simulink library "Heart_Signal_Processing_Library"  (R2021b)
settings: Solver=VariableStepAuto  StartTime=0.0  StopTime=10.0  RelTol=1e-3
undefined symbols (not defined in the file): sampleTime
libraries: coefficientsOfTunableBandpassFilter x10, simulink x2, dspindex x1
Description:
  | This library contains the subsystems that can be used to create the Pan-Tompkin algorithm and the Subsystems necessary for Non_invasive
  | Blood Pressure Signal Processing.
  | 
  | The lowpassFilter and the highpassFilter can be cascaded to create a first-order bandpass filter,
  | similar to that of the one used in the Pan-Tompkin Algorithm.
  | 
  | The tunableBandpassFilter is a second order bandpass filter with tunable quality factor and center frequency settings,
  | that can be used as a drop-in replacement to the cascaded lowpassFilter and highpassFilter.
  | 
  | The purpose of the bandpass filter is to attenuate the lower frequency and higher frequency components of the ecg signal, while
  | allowing the frequency of the QRS signal component to pass as an output.
  | 
  | The derivative filter is meant to be placed after a bandpass filter, and is designed to further amplify the QRS wave magnitude
  | since the QRS wave's rate of change is much larger than that of the remaining frequency components' magnitude.
  | 
  | The movingAvg (moving average) filter is designed to be placed after a squaring function (which should have been placed right after the derivative filter),
  | and is a done so that the area where the QRS is present is expanded in regards to timespan.
  | 
  | The tresholdQRS is a block that is used at two different locations in the Pan-Tompkin Algorithm.
  | The first location this block is used is right after the chosen bandpass filter and right before a delay that is placed to sync the output
  | of the first thresholdQRS with that of the second thresholdQRS. The signal that comes out of the delay is placed through an AND gate
  | with the signal that comes out of the second delay. This results in a detected QRS. The second thresholdQRS is to be placed after the movingAvg.
  | Independelty, both thresholdQRS output a possible QRS detection as a value of 1, these values, especially the one out of the first threshold,
  | are likely to contain false positives which is why they are synced and compared using AND logic.
  | 
  | The bandpassStartupTimer acts as a temporary buffer between the first 0.5 seconds of the chosen bandpass and the derivative filters.
  | Outputs 0 prior to the 0.5 seconds, and then passes the bandpass filter otuput into the derivative filter after the 0.5 seconds. This component
  | helps eliminate the possiblility of false negatives caused by an abnormally high signal threshold initial values that could occur prior to 0.5 seconds.
  | 
  | The QRS_startupTimer acts as a temporary buffer right before the final QRS detection output. Any value prior to 3.6 seconds is set to 0.
  | After 3.6 seconds, the intended confirmed QRS values are allowed through. This buffer helps prevent false positives caused during the
  | initialization of the system prior to 3.6 seconds. Note: The last known false positives occur before 2 seconds, but 3.6 seconds allows for an
  | addtional 80% margin of error.
settings Model: Creator=wallyproenza  LastModifiedBy=wallyproenza

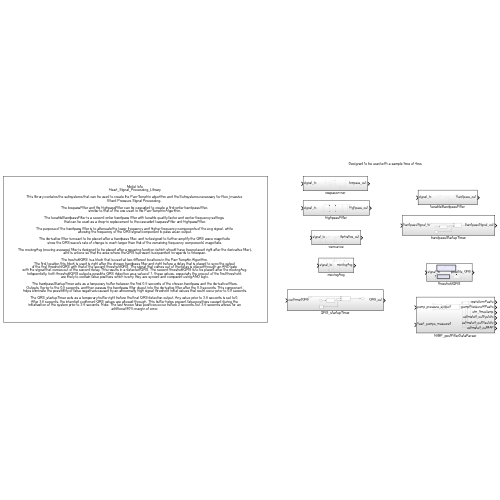
[thumbnail: Simulink's stored preview of the top-level diagram]
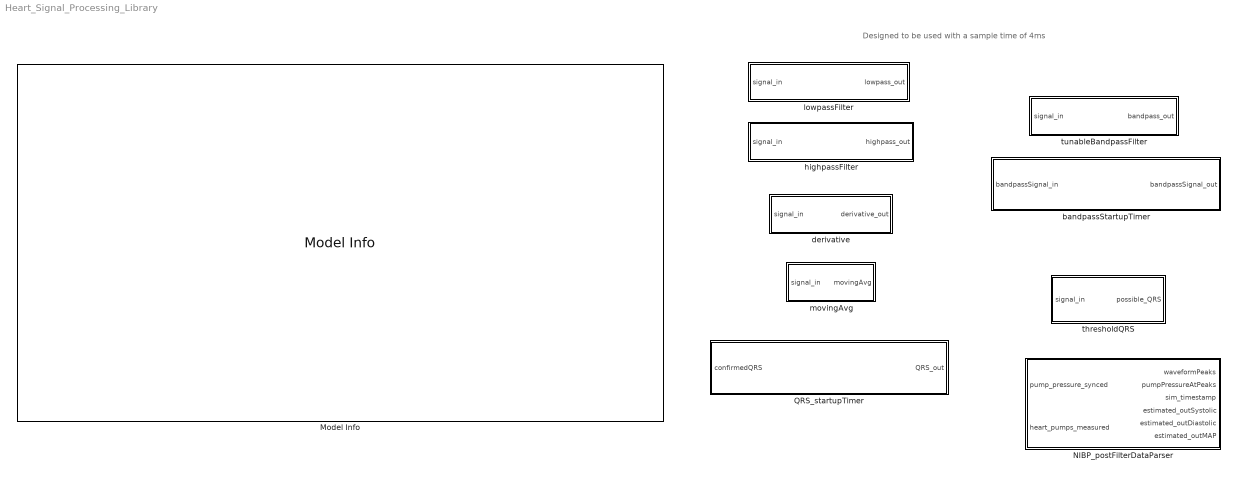
== system Heart_Signal_Processing_Library ==
  note: Designed to be used with a sample time of 4ms
  Model Info : simulink/Model-Wide Utilities/Model Info  Frame=on  DisplayStringWithTags=|  HorizontalTextAlignment=Center  LeftAlignmentValue=0.5
      | Model Info
      | %<ModelName>
      | 
      | %<Description>
  NIBP_postFilterDataParser : Subsystem
  QRS_startupTimer : Subsystem  Description=|
      | The QRS_startupTimer acts as a temporary buffer right before the final QRS detection output. Any value prior to 3.6 seconds is set to 0. 
      | After 3.6 seconds, the intended confirmed QRS values are allowed through. This buffer helps prevent false positives caused during the 
      | initialization of the system prior to 3.6 seconds. Note: The last known false positives occur before 2 seconds, but 3.6 seconds allows for an 
      | addtional 80% margin of error.
  bandpassStartupTimer : Subsystem  Description=|
      | The bandpassStartupTimer acts as a temporary buffer between the first 0.5 seconds of the chosen bandpass and the derivative filters.
      | Outputs 0 prior to the 0.5 seconds, and then passes the bandpass filter otuput into the derivative filter after the 0.5 seconds. This component 
      | helps eliminate the possiblility of false negatives caused by an abnormally high signal threshold initial values that could occur prior to 0.5 seconds.
  derivative : Subsystem  Description=|
      | The derivative filter is meant to be placed after a bandpass filter, and is designed to further amplify the QRS wave 
      | magnitude since the QRS wave's rate of change is much larger than that of the remaining frequency components' 
      | magnitude.
  highpassFilter : Subsystem  Description=|
      | Highpass filter described by the following difference equation:
      | y[n] = - (1/32)*x[n] + x[n-16] - x [n - 17] + (1/32)*x[n-32] + y[n-1]
  lowpassFilter : Subsystem  Description=|
      | Lowpass filter described by the below difference equation:
      | y[n] = (1/36)*(x[n] - 2x[n-6] + x[n-12]) + 2y[n-1] - y[n-2]
  movingAvg : Subsystem  Description=|
      | The movingAvg (moving average) filter is designed to be placed after a squaring function (which should have been placed right after the derivative filter),
      | and is a done so that the area where the QRS is present is expanded in regards to timespan. 
      | 
      | The moving average filter takes the average of the most recent 38 samples. This is implemented with a running sum of the most recent 38 samples 
      | with the 39th oldest sample subtracted whenever a new sample is introduced to the sum. Then the sum is divided by 38.
  thresholdQRS : Subsystem  Description=|
      | The tresholdQRS is a block that is used at two different locations in the Pan-Tompkin Algorithm. 
      | The first location this block is used is right after the chosen bandpass filter and right before a delay that is placed to sync the output 
      | of the first thresholdQRS with that of the second thresholdQRS. The signal that comes out of the delay is placed through an AND gate 
      | with the signal that comes out of the second delay. This results in a detected QRS. The second thresholdQRS is to be placed after the movingAvg.
      | Independelty, both thresholdQRS output a possible QRS detection as a value of 1, these values, especially the one out of the first threshold, 
      | are likely to contain false positives which is why they are synced and compared using AND logic.
  tunableBandpassFilter : Subsystem  Description=|
      | Bandpass Filter described by the following diference equation in terms of tunable centerFrequency f_o and qualityFactor Q:
      | y[n]=1/(250*10^3+π*10^3*f_o/Q  +4π^2 f_o^2 )*(π*10^3*f_o/Q x[n]  − π*10^3*f_o/Q x[n−2]  −(250*10^3−π*10^3*f_o/Q  +4π^2 f_o^2 )y[n−2]−2*(4π^2 f_o^2  −250*10^3 )y[n−1])
      | 
      | 
      | For simplicity, let constants A, B, and C be subsystems that contain the corresponding defintiions of the coefficients:
      | y[n] = 1/(A+ B + C ) * {Bx[n]  − Bx[n−2]  − (A − B + C )y[n−2]− 2*(C  − A)y[n−1]}
      | 
      | where,
      | A = 250*10^3
      | B = π*10^3*f_o/Q  
      | C = 4π^2 f_o^2

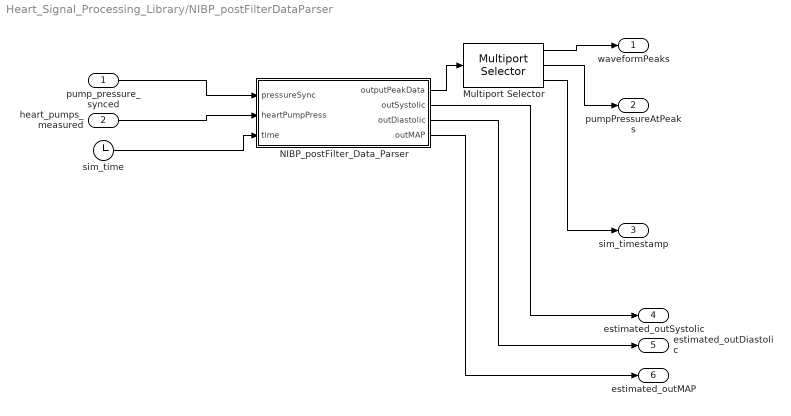
== system Heart_Signal_Processing_Library/NIBP_postFilterDataParser ==
  pump_pressure_synced : Inport
  heart_pumps_measured : Inport  Port=2
  Multiport Selector : dspindex/Multiport Selector  rowsOrCols=Columns  idxCellArray={ 1, 2, 3}  idxErrMode=Clip Index
  NIBP_postFilter_Data_Parser : MATLAB Function  TreatAsAtomicUnit=on
  sim_time : Clock
  waveformPeaks : Outport
  pumpPressureAtPeaks : Outport  Port=2
  sim_timestamp : Outport  Port=3
  estimated_outSystolic : Outport  Port=4
  estimated_outDiastolic : Outport  Port=5
  estimated_outMAP : Outport  Port=6
  wires:
  heart_pumps_measured/1 -> NIBP_postFilter_Data_Parser/2(heartPumpPress)
  Multiport Selector/3 -> sim_timestamp/1
  NIBP_postFilter_Data_Parser/3(outDiastolic) -> estimated_outDiastolic/1
  NIBP_postFilter_Data_Parser/4(outMAP) -> estimated_outMAP/1
  pump_pressure_synced/1 -> NIBP_postFilter_Data_Parser/1(pressureSync)
  Multiport Selector/1 -> waveformPeaks/1
  sim_time/1 -> NIBP_postFilter_Data_Parser/3(time)
  NIBP_postFilter_Data_Parser/2(outSystolic) -> estimated_outSystolic/1
  Multiport Selector/2 -> pumpPressureAtPeaks/1
  NIBP_postFilter_Data_Parser/1(outputPeakData) -> Multiport Selector/1

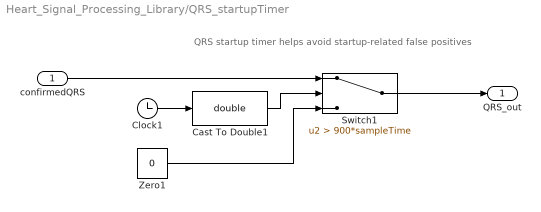
== system Heart_Signal_Processing_Library/QRS_startupTimer ==
  note: QRS startup timer helps avoid startup-related false positives
  confirmedQRS : Inport
  Cast To Double1 : DataTypeConversion  OutDataTypeStr=double
  Clock1 : Clock
  Switch1 : Switch  Criteria=u2 > Threshold  Threshold=900*sampleTime
  Zero1 : Constant  Value=0  OutDataTypeStr=Inherit: Inherit via back propagation
  QRS_out : Outport
  wires:
  confirmedQRS/1 -> Switch1/1
  Zero1/1 -> Switch1/3
  Cast To Double1/1 -> Switch1/2
  Switch1/1 -> QRS_out/1
  Clock1/1 -> Cast To Double1/1

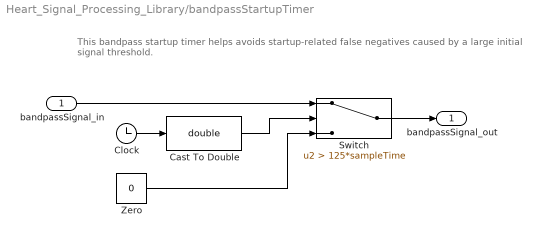
== system Heart_Signal_Processing_Library/bandpassStartupTimer ==
  note: This bandpass startup timer helps avoids startup-related false negatives
      | caused by a large initial signal threshold.
  bandpassSignal_in : Inport
  Cast To Double : DataTypeConversion  OutDataTypeStr=double
  Clock : Clock
  Switch : Switch  Criteria=u2 > Threshold  Threshold=125*sampleTime
  Zero : Constant  Value=0  OutDataTypeStr=Inherit: Inherit via back propagation
  bandpassSignal_out : Outport
  wires:
  Cast To Double/1 -> Switch/2
  Switch/1 -> bandpassSignal_out/1
  bandpassSignal_in/1 -> Switch/1
  Zero/1 -> Switch/3
  Clock/1 -> Cast To Double/1

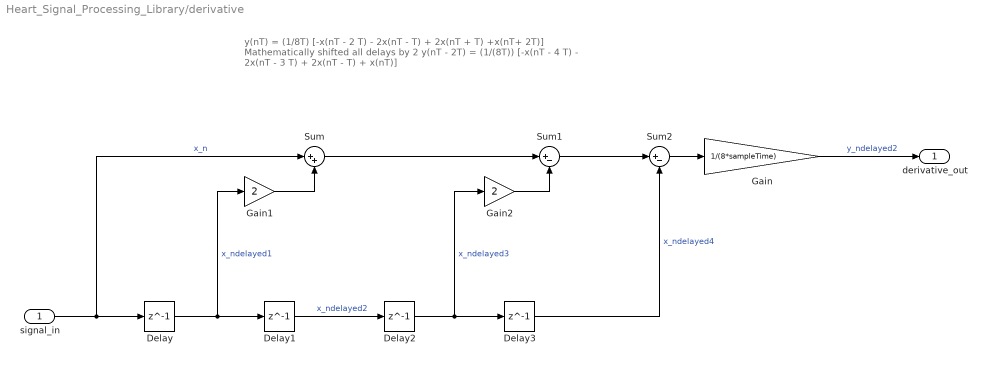
== system Heart_Signal_Processing_Library/derivative ==
  note: y(nT) = (1/8T) [-x(nT - 2 T) - 2x(nT - T) + 2x(nT + T) +x(nT+ 2T)]
      |
      | Mathematically shifted all delays by 2
      |
      | y(nT - 2T) = (1/(8T)) [-x(nT - 4 T) - 2x(nT - 3 T) + 2x(nT - T) + x(nT)]
  signal_in : Inport
  Delay{,1..3} (4 alike) : Delay  DelayLength=1  InitialCondition=0
  Gain : Gain  Gain=1/(8*sampleTime)
  Gain1 : Gain  Gain=2
  Gain2 : Gain  Gain=2
  Sum : Sum  Inputs=|++
  Sum1 : Sum  Inputs=|+-
  Sum2 : Sum  Inputs=|+-
  derivative_out : Outport
  wires:
  Gain/1 -> derivative_out/1  "y_ndelayed2"
  signal_in/1 -> Sum/1, Delay/1  "x_n"
  Delay/1 -> Gain1/1, Delay1/1  "x_ndelayed1"
  Delay1/1 -> Delay2/1  "x_ndelayed2"
  Delay2/1 -> Gain2/1, Delay3/1  "x_ndelayed3"
  Delay3/1 -> Sum2/2  "x_ndelayed4"
  Gain1/1 -> Sum/2
  Gain2/1 -> Sum1/2
  Sum/1 -> Sum1/1
  Sum1/1 -> Sum2/1
  Sum2/1 -> Gain/1

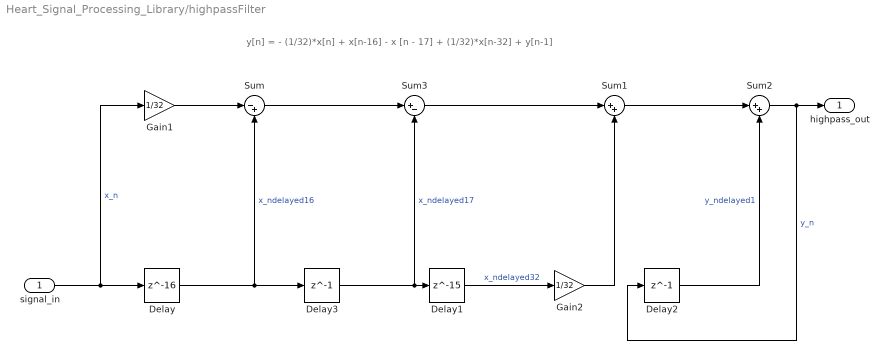
== system Heart_Signal_Processing_Library/highpassFilter ==
  note: y[n] = - (1/32)*x[n] + x[n-16] - x [n - 17] + (1/32)*x[n-32] + y[n-1]
  signal_in : Inport
  Delay : Delay  DelayLength=16  InitialCondition=0
  Delay1 : Delay  DelayLength=15  InitialCondition=0
  Delay2 : Delay  DelayLength=1  InitialCondition=0
  Delay3 : Delay  DelayLength=1  InitialCondition=0
  Gain1 : Gain  Gain=1/32
  Gain2 : Gain  Gain=1/32
  Sum : Sum  Inputs=|-+
  Sum1 : Sum  Inputs=|++
  Sum2 : Sum  Inputs=|++
  Sum3 : Sum  Inputs=|+-
  highpass_out : Outport
  wires:
  signal_in/1 -> Gain1/1, Delay/1  "x_n"
  Delay/1 -> Delay3/1, Sum/2  "x_ndelayed16"
  Delay1/1 -> Gain2/1  "x_ndelayed32"
  Sum1/1 -> Sum2/1
  Delay2/1 -> Sum2/2  "y_ndelayed1"
  Sum2/1 -> Delay2/1, highpass_out/1  "y_n"
  Gain1/1 -> Sum/1
  Delay3/1 -> Delay1/1, Sum3/2  "x_ndelayed17"
  Sum/1 -> Sum3/1
  Sum3/1 -> Sum1/1
  Gain2/1 -> Sum1/2

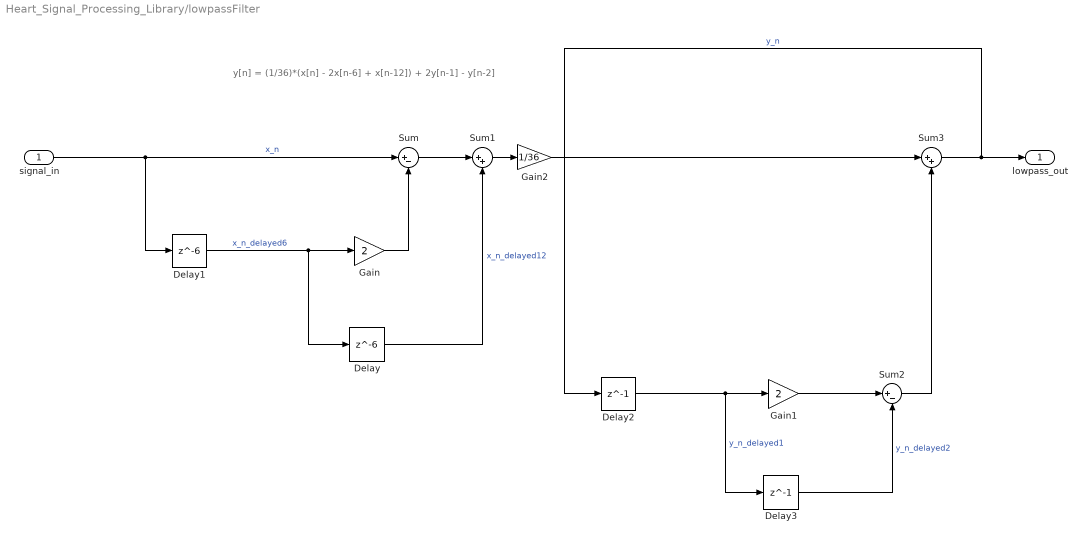
== system Heart_Signal_Processing_Library/lowpassFilter ==
  note: y[n] = (1/36)*(x[n] - 2x[n-6] + x[n-12]) + 2y[n-1] - y[n-2]
  signal_in : Inport
  Delay : Delay  DelayLength=6  InitialCondition=0
  Delay1 : Delay  DelayLength=6  InitialCondition=0
  Delay2 : Delay  DelayLength=1  InitialCondition=0
  Delay3 : Delay  DelayLength=1  InitialCondition=0
  Gain : Gain  Gain=2
  Gain1 : Gain  Gain=2
  Gain2 : Gain  Gain=1/36
  Sum : Sum  Inputs=|+-
  Sum1 : Sum  Inputs=|++
  Sum2 : Sum  Inputs=|+-
  Sum3 : Sum  Inputs=|++
  lowpass_out : Outport
  wires:
  signal_in/1 -> Delay1/1, Sum/1  "x_n"
  Delay1/1 -> Gain/1, Delay/1  "x_n_delayed6"
  Gain/1 -> Sum/2
  Delay/1 -> Sum1/2  "x_n_delayed12"
  Sum/1 -> Sum1/1
  Sum1/1 -> Gain2/1
  Delay2/1 -> Delay3/1, Gain1/1  "y_n_delayed1"
  Gain1/1 -> Sum2/1
  Delay3/1 -> Sum2/2  "y_n_delayed2"
  Sum2/1 -> Sum3/2
  Sum3/1 -> lowpass_out/1, Delay2/1  "y_n"
  Gain2/1 -> Sum3/1

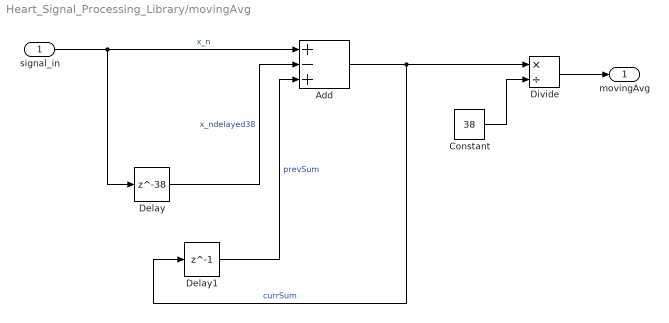
== system Heart_Signal_Processing_Library/movingAvg ==
  signal_in : Inport
  Add : Sum  Inputs=+-+
  Constant : Constant  Value=38
  Delay : Delay  DelayLength=38  InitialCondition=0
  Delay1 : Delay  DelayLength=1  InitialCondition=0
  Divide : Product  Inputs=*/
  movingAvg : Outport
  wires:
  Constant/1 -> Divide/2
  Divide/1 -> movingAvg/1
  signal_in/1 -> Delay/1, Add/1  "x_n"
  Delay/1 -> Add/2  "x_ndelayed38"
  Add/1 -> Divide/1, Delay1/1  "currSum"
  Delay1/1 -> Add/3  "prevSum"

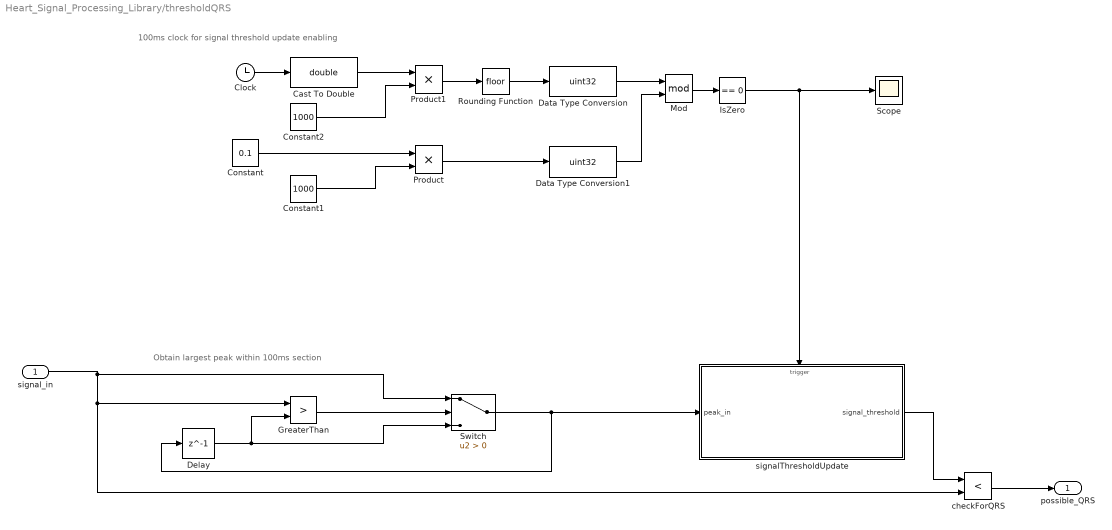
== system Heart_Signal_Processing_Library/thresholdQRS ==
  note: Obtain largest peak within 100ms section
  note: 100ms clock for signal threshold update enabling
  signal_in : Inport
  Cast To Double : DataTypeConversion  OutDataTypeStr=double
  Clock : Clock
  Constant : Constant  Value=0.1
  Constant1 : Constant  Value=1000
  Constant2 : Constant  Value=1000
  Data Type Conversion : DataTypeConversion  OutDataTypeStr=uint32
  Data Type Conversion1 : DataTypeConversion  OutDataTypeStr=uint32
  Delay : Delay  DelayLength=1  InitialCondition=0
  GreaterThan : RelationalOperator  Operator=>  OutDataTypeStr=boolean  RndMeth=Simplest
  IsZero : simulink/Logic and Bit Operations/Compare To Zero  relop===  OutDataTypeStr=boolean
  Mod : Math  Operator=mod  SaturateOnIntegerOverflow=on
  Product : Product
  Product1 : Product
  Rounding Function : Rounding
  Scope : Scope
  Switch : Switch  Criteria=u2 > Threshold
  checkForQRS : RelationalOperator  Operator=<  OutDataTypeStr=boolean  RndMeth=Simplest
  signalThresholdUpdate : Subsystem
  possible_QRS : Outport
  wires:
  signal_in/1 -> checkForQRS/2, GreaterThan/1, Switch/1
  signalThresholdUpdate/1(signal_threshold) -> checkForQRS/1
  Rounding Function/1 -> Data Type Conversion/1
  Constant/1 -> Product/1
  Product/1 -> Data Type Conversion1/1
  Constant1/1 -> Product/2
  Constant2/1 -> Product1/2
  Clock/1 -> Cast To Double/1
  Product1/1 -> Rounding Function/1
  Data Type Conversion1/1 -> Mod/2
  Data Type Conversion/1 -> Mod/1
  Mod/1 -> IsZero/1
  IsZero/1 -> signalThresholdUpdate/Trigger, Scope/1
  Cast To Double/1 -> Product1/1
  checkForQRS/1 -> possible_QRS/1
  GreaterThan/1 -> Switch/2
  Switch/1 -> Delay/1, signalThresholdUpdate/1(peak_in)
  Delay/1 -> Switch/3, GreaterThan/2

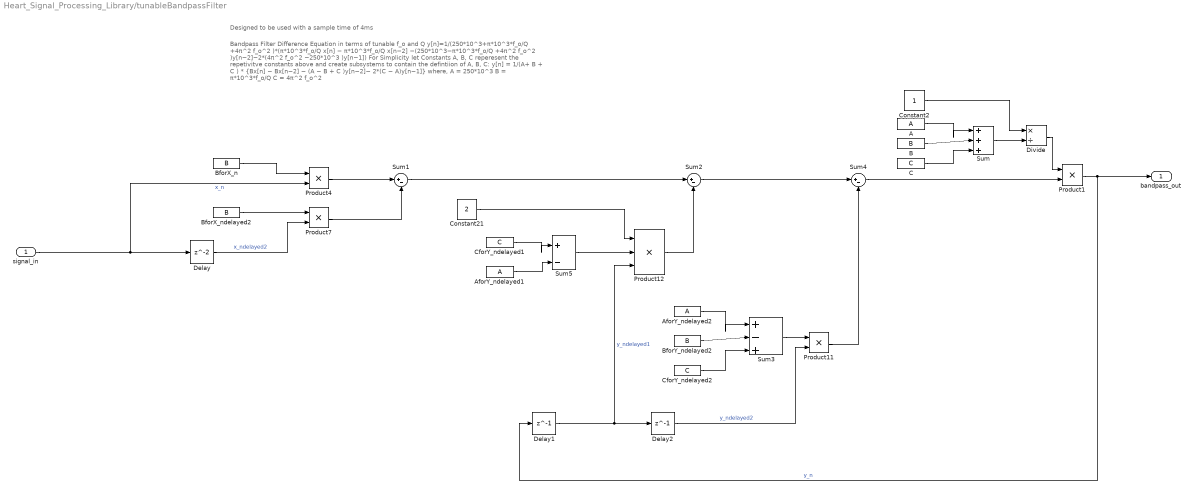
== system Heart_Signal_Processing_Library/tunableBandpassFilter ==
  note: Bandpass Filter Difference Equation in terms of tunable f_o and Q
      |
      | y[n]=1/(250*10^3+π*10^3*f_o/Q +4π^2 f_o^2 )*(π*10^3*f_o/Q x[n] − π*10^3*f_o/Q x[n−2] −(250*10^3−π*10^3*f_o/Q +4π^2 f_o^2 )y[n−2]−2*(4π^2 f_o^2 −250*10^3 )y[n−1])
      |
      | For Simplicity let Constants A, B, C reperesent the repetivitve constants above and create subsystems to contain the defintiion of A, B, C:
      |
      | y[n] = 1/(A+ B + C ) * {Bx[n] − Bx[n−2] − (A − B + C )y[n−2]− 2*(C − A)y[n−1]}
      |
      | where,
      | A = 250*10^3
      | B = π*10^3*f_o/Q
      | C = 4π^2 f_o^2
  note: Designed to be used with a sample time of 4ms
  signal_in : Inport
  A : coefficientsOfTunableBandpassFilter/A  SystemSampleTime=-1  VariantActivationTime=update diagram  Latency=0  AutoFrameSizeCalculation=off
  AforY_ndelayed1 : coefficientsOfTunableBandpassFilter/A  SystemSampleTime=-1  VariantActivationTime=update diagram  Latency=0  AutoFrameSizeCalculation=off
  AforY_ndelayed2 : coefficientsOfTunableBandpassFilter/A  SystemSampleTime=-1  VariantActivationTime=update diagram  Latency=0  AutoFrameSizeCalculation=off
  B : coefficientsOfTunableBandpassFilter/B  SystemSampleTime=-1  VariantActivationTime=update diagram  Latency=0  AutoFrameSizeCalculation=off
  BforX_n : coefficientsOfTunableBandpassFilter/B  SystemSampleTime=-1  VariantActivationTime=update diagram  Latency=0  AutoFrameSizeCalculation=off
  BforX_ndelayed2 : coefficientsOfTunableBandpassFilter/B  SystemSampleTime=-1  VariantActivationTime=update diagram  Latency=0  AutoFrameSizeCalculation=off
  BforY_ndelayed2 : coefficientsOfTunableBandpassFilter/B  SystemSampleTime=-1  VariantActivationTime=update diagram  Latency=0  AutoFrameSizeCalculation=off
  C : coefficientsOfTunableBandpassFilter/C  SystemSampleTime=-1  VariantActivationTime=update diagram  Latency=0  AutoFrameSizeCalculation=off
  CforY_ndelayed1 : coefficientsOfTunableBandpassFilter/C  SystemSampleTime=-1  VariantActivationTime=update diagram  Latency=0  AutoFrameSizeCalculation=off
  CforY_ndelayed2 : coefficientsOfTunableBandpassFilter/C  SystemSampleTime=-1  VariantActivationTime=update diagram  Latency=0  AutoFrameSizeCalculation=off
  Constant2 : Constant
  Constant21 : Constant  Value=2
  Delay : Delay  InitialCondition=0
  Delay1 : Delay  DelayLength=1  InitialCondition=0
  Delay2 : Delay  DelayLength=1  InitialCondition=0
  Divide : Product  Inputs=*/
  Product{1,4,7,11} (4 alike) : Product
  Product12 : Product  Inputs=3
  Sum : Sum  Inputs=|+++
  Sum{1..2,4..5} (4 alike) : Sum  Inputs=|+-
  Sum3 : Sum  Inputs=|+-+
  bandpass_out : Outport
  wires:
  signal_in/1 -> Product4/2, Delay/1  "x_n"
  Delay1/1 -> Product12/3, Delay2/1  "y_ndelayed1"
  Product1/1 -> Delay1/1, bandpass_out/1  "y_n"
  Constant2/1 -> Divide/1
  Sum/1 -> Divide/2
  Divide/1 -> Product1/1
  Product4/1 -> Sum1/1
  Product7/1 -> Sum1/2
  Delay/1 -> Product7/2  "x_ndelayed2"
  Sum1/1 -> Sum2/1
  Sum3/1 -> Product11/1
  Product11/1 -> Sum4/2
  Delay2/1 -> Product11/2  "y_ndelayed2"
  Sum4/1 -> Product1/2
  Sum2/1 -> Sum4/1
  Product12/1 -> Sum2/2
  Constant21/1 -> Product12/1
  Sum5/1 -> Product12/2
  A/1 -> Sum/1
  B/1 -> Sum/2
  C/1 -> Sum/3
  BforX_n/1 -> Product4/1
  BforX_ndelayed2/1 -> Product7/1
  AforY_ndelayed1/1 -> Sum5/2
  CforY_ndelayed1/1 -> Sum5/1
  AforY_ndelayed2/1 -> Sum3/1
  BforY_ndelayed2/1 -> Sum3/2
  CforY_ndelayed2/1 -> Sum3/3

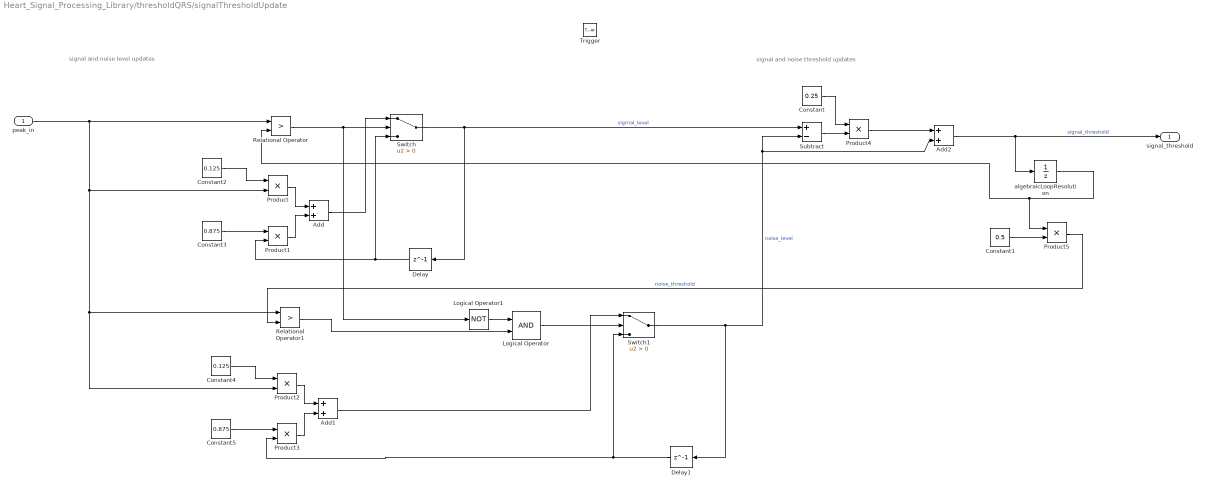
== system Heart_Signal_Processing_Library/thresholdQRS/signalThresholdUpdate ==
  note: signal and noise threshold updates
  note: signal and noise level updates
  peak_in : Inport
  Trigger : TriggerPort  VariantControl=(inherit)  PortDimensions=1
  Add : Sum
  Add1 : Sum
  Add2 : Sum
  Constant : Constant  Value=0.25
  Constant1 : Constant  Value=0.5
  Constant2 : Constant  Value=0.125
  Constant3 : Constant  Value=0.875
  Constant4 : Constant  Value=0.125
  Constant5 : Constant  Value=0.875
  Delay : Delay  DelayLength=1  InitialCondition=0
  Delay1 : Delay  DelayLength=1  InitialCondition=0
  Logical Operator : Logic  IconShape=distinctive  AllPortsSameDT=off  OutDataTypeStr=boolean
  Logical Operator1 : Logic  Operator=NOT  IconShape=distinctive  AllPortsSameDT=off  OutDataTypeStr=boolean
  Product{,1..5} (6 alike) : Product
  Relational Operator : RelationalOperator  Operator=>  OutDataTypeStr=boolean  RndMeth=Simplest
  Relational Operator1 : RelationalOperator  Operator=>  OutDataTypeStr=boolean  RndMeth=Simplest
  Subtract : Sum  Inputs=+-
  Switch : Switch  Criteria=u2 > Threshold
  Switch1 : Switch  Criteria=u2 > Threshold
  algebraicLoopResolution : UnitDelay  SampleTime=-1  HasFrameUpgradeWarning=on
  signal_threshold : Outport
  wires:
  Constant5/1 -> Product3/1
  Product3/1 -> Add1/2
  Add/1 -> Switch/1
  Product2/1 -> Add1/1
  Switch1/1 -> Delay1/1, Add2/2, Subtract/2  "noise_level"
  Product/1 -> Add/1
  Constant2/1 -> Product/1
  Constant1/1 -> Product5/2
  Add2/1 -> algebraicLoopResolution/1, signal_threshold/1  "signal_threshold"
  Product4/1 -> Add2/1
  Logical Operator/1 -> Switch1/2
  Constant/1 -> Product4/1
  peak_in/1 -> Relational Operator/1, Product/2, Relational Operator1/1, Product2/2
  Delay1/1 -> Product3/2, Switch1/3
  Logical Operator1/1 -> Logical Operator/1
  Constant4/1 -> Product2/1
  Delay/1 -> Switch/3, Product1/2
  Product1/1 -> Add/2
  Add1/1 -> Switch1/1
  Switch/1 -> Delay/1, Subtract/1  "sigmal_level"
  Constant3/1 -> Product1/1
  Relational Operator/1 -> Logical Operator1/1, Switch/2
  Product5/1 -> Relational Operator1/2  "noise_threshold"
  Subtract/1 -> Product4/2
  Relational Operator1/1 -> Logical Operator/2
  algebraicLoopResolution/1 -> Product5/1, Relational Operator/2

== matlab function Heart_Signal_Processing_Library/NIBP_postFilterDataParser/NIBP_postFilter_Data_Parser ==
  data: pressureSync input; outputPeakData output; heartPumpPress input; time input; outSystolic output; outDiastolic output; outMAP output
function [outputPeakData, outSystolic, outDiastolic, outMAP] = ...
    fcn(pressureSync, heartPumpPress, time)
INCLINE = 0;
DECLINE = 1;
CONSTANT = 2;
persistent index
    if isempty(index)
        index = 1;
    end

persistent peaks
    if isempty(peaks)
        peaks = zeros(30,3);
    end
persistent prevHeartPumpPress
    if isempty(prevHeartPumpPress)
         prevHeartPumpPress = 0;
    end
persistent prevSlope
    if isempty(prevSlope)
        prevSlope = CONSTANT;
    end
    

slope = CONSTANT;   
if(heartPumpPress > prevHeartPumpPress)
    slope = INCLINE;
elseif(heartPumpPress < prevHeartPumpPress)
    slope = DECLINE;
else
    slope = CONSTANT;
end

local_max = 0;
if(prevSlope == INCLINE && slope == DECLINE)
    %Local Max found
    local_max = 1;
    updatePrevSlope = 1;
elseif(prevSlope == DECLINE && slope == INCLINE)
    %Local Min found instead
    local_max = 0;
    updatePrevSlope = 1;
elseif((prevSlope == DECLINE || prevSlope == INCLINE) && slope == CONSTANT)
    %do not update prevSlope
    updatePrevSlope = 0;
else
    updatePrevSlope = DECLINE;
end

if(updatePrevSlope == 1)
prevSlope = slope;
end


if(local_max == 1 && index <= 30)
        peaks(index,1) = heartPumpPress;
        peaks(index,2) = pressureSync;
        peaks(index,3) = time;
        index = index + 1;
end
    
diastolic = 0;
i = 1;
while (diastolic == 0 && i <= 30 && time > 59.975)
    if ((peaks((31-i),1)) ~= 0)
    diastolic = (peaks((31-i),2));
    end
    i = i + 1;
end
prevHeartPumpPress = heartPumpPress;
systolic = peaks(1,2);
MAP = (1/3) * systolic + (2/3) * diastolic; 

outDiastolic = diastolic;
outSystolic = systolic;
outMAP = MAP;
outputPeakData = peaks;
end
